simulink model "bf16_mac_new"  (R2022b)
settings: Solver=VariableStepAuto  StartTime=0.0  StopTime=10.0  RelTol=1e-3
libraries: hdlsllib x116, simulink x24
(part 1 of 2)
settings Model: Creator=zishu wu  LastModifiedBy=zishu wu

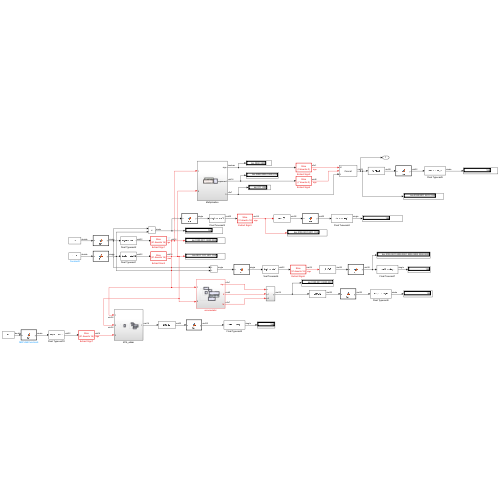
[thumbnail: Simulink's stored preview of the top-level diagram]
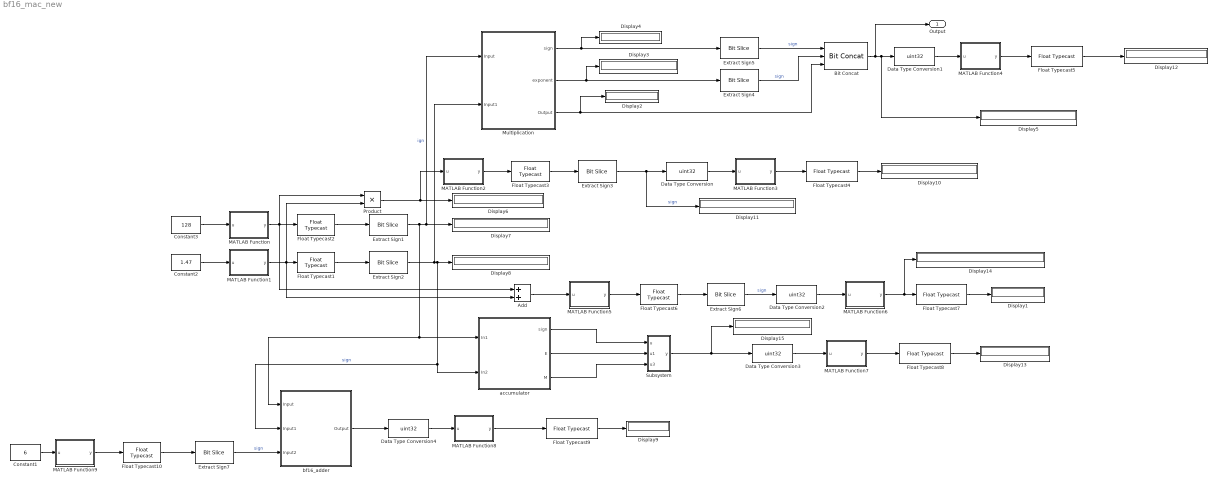
== system bf16_mac_new ==
  Add : Sum
  Bit Concat : hdlsllib/Logic and Bit Operations/Bit Concat  numInputs=3
  Constant1 : Constant  Value=6  OutDataTypeStr=double
  Constant2 : Constant  Value=1.47  OutDataTypeStr=double
  Constant3 : Constant  Value=128  OutDataTypeStr=double  SampleTime=1.5625
  Data Type Conversion{,1..4} (5 alike) : DataTypeConversion  OutDataTypeStr=uint32  SaturateOnIntegerOverflow=off  RndMeth=Floor
  Display{1..15} (15 alike) : Display
      settings: Format=binary (Stored Integer)
  Extract Sign{1..3,6..7} (5 alike) : hdlsllib/Logic and Bit Operations/Bit Slice  lidx=31  ridx=16
  Extract Sign4 : hdlsllib/Logic and Bit Operations/Bit Slice  lidx=7  ridx=0
  Extract Sign5 : hdlsllib/Logic and Bit Operations/Bit Slice  lidx=0  ridx=0
  Float Typecast{1..10} (10 alike) : FloatTypecast
  MATLAB Function : MATLAB Function  TreatAsAtomicUnit=on
  MATLAB Function1 : MATLAB Function  TreatAsAtomicUnit=on
  MATLAB Function2 : MATLAB Function  TreatAsAtomicUnit=on
  MATLAB Function3 : MATLAB Function  TreatAsAtomicUnit=on
  MATLAB Function4 : MATLAB Function  TreatAsAtomicUnit=on
  MATLAB Function5 : MATLAB Function  TreatAsAtomicUnit=on
  MATLAB Function6 : MATLAB Function  TreatAsAtomicUnit=on
  MATLAB Function7 : MATLAB Function  TreatAsAtomicUnit=on
  MATLAB Function8 : MATLAB Function  TreatAsAtomicUnit=on
  MATLAB Function9 : MATLAB Function  TreatAsAtomicUnit=on
  Multiplication : Subsystem
  Product : Product
  Subsystem : Subsystem
  accumulator : Subsystem
  bf16_adder : Subsystem
  Output : Outport
  wires:
  Bit Concat/1 -> Output/1, Display5/1, Data Type Conversion1/1
  Multiplication/2(exponent) -> Extract Sign4/1, Display3/1
  Multiplication/1(sign) -> Display4/1, Extract Sign5/1
  Float Typecast2/1 -> Extract Sign1/1
  MATLAB Function/1(y) -> Add/1, Product/1, Float Typecast2/1
  MATLAB Function1/1(y) -> Add/2, Product/2, Float Typecast1/1
  Float Typecast1/1 -> Extract Sign2/1
  Extract Sign2/1 -> Multiplication/2(Input1), bf16_adder/2(Input1), accumulator/2(In2), Display8/1  "sign"
  Extract Sign1/1 -> Multiplication/1(Input), Display7/1, accumulator/1(In1), bf16_adder/1(Input)  "ign"
  Product/1 -> MATLAB Function2/1(u), Display6/1
  MATLAB Function2/1(y) -> Float Typecast3/1
  Float Typecast3/1 -> Extract Sign3/1
  Extract Sign3/1 -> Display11/1, Data Type Conversion/1  "sign"
  Extract Sign4/1 -> Bit Concat/2  "sign"
  Extract Sign5/1 -> Bit Concat/1  "sign"
  Data Type Conversion/1 -> MATLAB Function3/1(u)
  Float Typecast4/1 -> Display10/1
  Data Type Conversion1/1 -> MATLAB Function4/1(u)
  MATLAB Function3/1(y) -> Float Typecast4/1
  MATLAB Function4/1(y) -> Float Typecast5/1
  Float Typecast6/1 -> Extract Sign6/1
  MATLAB Function5/1(y) -> Float Typecast6/1
  Add/1 -> MATLAB Function5/1(u)
  MATLAB Function6/1(y) -> Display14/1, Float Typecast7/1
  Data Type Conversion2/1 -> MATLAB Function6/1(u)
  Float Typecast7/1 -> Display1/1
  Extract Sign6/1 -> Data Type Conversion2/1  "sign"
  Float Typecast8/1 -> Display13/1
  Data Type Conversion3/1 -> MATLAB Function7/1(u)
  MATLAB Function7/1(y) -> Float Typecast8/1
  Subsystem/1(y) -> Data Type Conversion3/1, Display15/1
  Constant3/1 -> MATLAB Function/1(u)
  Constant2/1 -> MATLAB Function1/1(u)
  Float Typecast5/1 -> Display12/1
  MATLAB Function8/1(y) -> Float Typecast9/1
  Data Type Conversion4/1 -> MATLAB Function8/1(u)
  Float Typecast9/1 -> Display9/1
  bf16_adder/1(Output) -> Data Type Conversion4/1
  accumulator/1(sign) -> Subsystem/1(u)
  accumulator/2(E) -> Subsystem/2(u1)
  accumulator/3(M) -> Subsystem/3(u3)
  Multiplication/3(Output) -> Display2/1, Bit Concat/3
  Float Typecast10/1 -> Extract Sign7/1
  MATLAB Function9/1(y) -> Float Typecast10/1
  Extract Sign7/1 -> bf16_adder/3(Input2)  "sign"
  Constant1/1 -> MATLAB Function9/1(u)

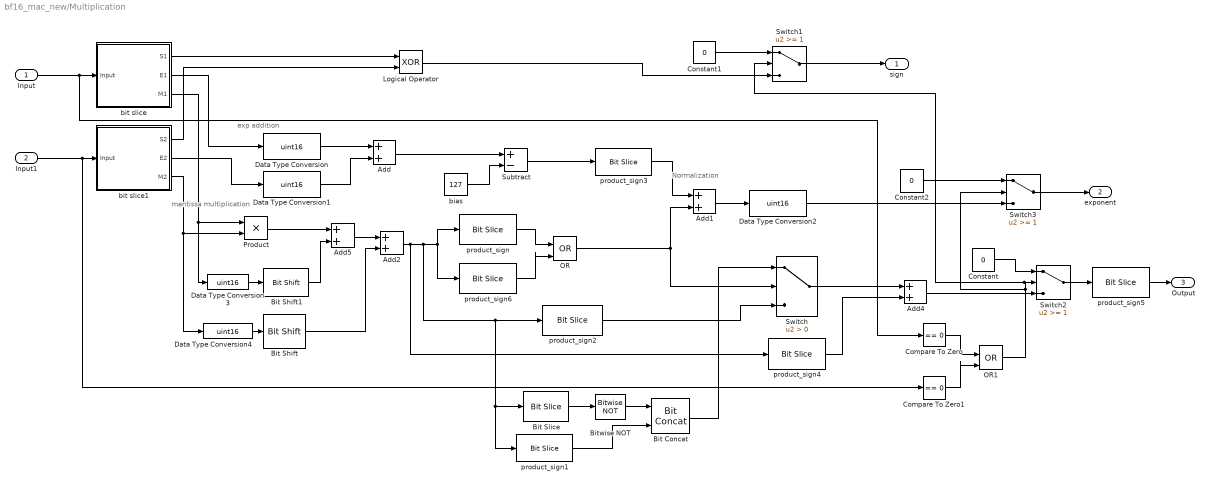
== system bf16_mac_new/Multiplication ==
  note: mantissa multiplication
  note: Normalization
  note: exp addition
  Input : Inport
  Input1 : Inport  Port=2
  Add{,2,4..5} (4 alike) : Sum  AccumDataTypeStr=uint16
  Add1 : Sum
  Bit Concat : hdlsllib/Logic and Bit Operations/Bit Concat  numInputs=2
  Bit Shift : hdlsllib/Logic and Bit Operations/Bit Shift  mode=Shift Left Logical  N=7
  Bit Shift1 : hdlsllib/Logic and Bit Operations/Bit Shift  mode=Shift Left Logical  N=7
  Bit Slice : hdlsllib/Logic and Bit Operations/Bit Slice  lidx=14  ridx=14
  Bitwise NOT : simulink/Logic and Bit Operations/Bitwise Operator  logicop=NOT  UseBitMask=off  BitMask=bin2dec('11011001')  BitMaskRealWorld=Stored Integer
      settings: LibrarySourceBlock=|
      | simulink/Quick Insert/Logic and Bit
      | Operations/Bitwise NOT
  Compare To Zero : simulink/Logic and Bit Operations/Compare To Zero  relop===  OutDataTypeStr=boolean
  Compare To Zero1 : simulink/Logic and Bit Operations/Compare To Zero  relop===  OutDataTypeStr=boolean
  Constant : Constant  Value=0  OutDataTypeStr=uint8
  Constant1 : Constant  Value=0  OutDataTypeStr=boolean
  Constant2 : Constant  Value=0  OutDataTypeStr=uint16
  Data Type Conversion{,1..4} (5 alike) : DataTypeConversion  OutDataTypeStr=uint16  SaturateOnIntegerOverflow=off  RndMeth=Floor
  Logical Operator : Logic  Operator=XOR  AllPortsSameDT=off  OutDataTypeStr=boolean
  OR : Logic  Operator=OR  IconShape=distinctive  AllPortsSameDT=off  OutDataTypeStr=boolean
  OR1 : Logic  Operator=OR  IconShape=distinctive  AllPortsSameDT=off  OutDataTypeStr=boolean
  Product : Product  OutDataTypeStr=uint16
  Subtract : Sum  Inputs=+-
  Switch : Switch  Criteria=u2 > Threshold  SaturateOnIntegerOverflow=off  InputSameDT=off
  Switch1 : Switch  Threshold=1  SaturateOnIntegerOverflow=off  InputSameDT=off
  Switch2 : Switch  Threshold=1  SaturateOnIntegerOverflow=off  InputSameDT=off
  Switch3 : Switch  Threshold=1  SaturateOnIntegerOverflow=off  InputSameDT=off
  bias : Constant  Value=127  OutDataTypeStr=uint16
  bit slice : Subsystem
  bit slice1 : Subsystem
  product_sign : hdlsllib/Logic and Bit Operations/Bit Slice  lidx=15  ridx=15
  product_sign1 : hdlsllib/Logic and Bit Operations/Bit Slice  lidx=13  ridx=7
  product_sign2 : hdlsllib/Logic and Bit Operations/Bit Slice  lidx=13  ridx=6
  product_sign3 : hdlsllib/Logic and Bit Operations/Bit Slice  lidx=7  ridx=0
  product_sign4 : hdlsllib/Logic and Bit Operations/Bit Slice  lidx=0  ridx=0
  product_sign5 : hdlsllib/Logic and Bit Operations/Bit Slice  lidx=7  ridx=1
  product_sign6 : hdlsllib/Logic and Bit Operations/Bit Slice  lidx=14  ridx=14
  sign : Outport
  exponent : Outport  Port=2
  Output : Outport  Port=3
  wires:
  product_sign/1 -> OR/1
  Compare To Zero1/1 -> OR1/2
  Bitwise NOT/1 -> Bit Concat/1
  Add5/1 -> Add2/1
  Input/1 -> Compare To Zero/1, bit slice/1(Input)
  Product/1 -> Add5/1
  product_sign6/1 -> OR/2
  Switch/1 -> Add4/1
  Subtract/1 -> product_sign3/1
  Data Type Conversion4/1 -> Bit Shift/1
  bit slice1/1(S2) -> Logical Operator/2
  Input1/1 -> Compare To Zero1/1, bit slice1/1(Input)
  Add1/1 -> Data Type Conversion2/1
  Constant2/1 -> Switch3/1
  Switch1/1 -> sign/1
  Data Type Conversion/1 -> Add/1
  Bit Slice/1 -> Bitwise NOT/1
  Switch3/1 -> exponent/1
  product_sign3/1 -> Add1/1
  OR1/1 -> Switch1/2, Switch2/2, Switch3/2
  Constant1/1 -> Switch1/1
  Data Type Conversion1/1 -> Add/2
  Constant/1 -> Switch2/1
  Add2/1 -> product_sign4/1, product_sign1/1, Bit Slice/1, product_sign2/1, product_sign6/1, product_sign/1
  product_sign5/1 -> Output/1
  product_sign4/1 -> Add4/2
  Logical Operator/1 -> Switch1/3
  Bit Concat/1 -> Switch/1
  bias/1 -> Subtract/2
  Data Type Conversion2/1 -> Switch3/3
  OR/1 -> Add1/2, Switch/2
  Switch2/1 -> product_sign5/1
  bit slice/2(E1) -> Data Type Conversion/1
  Add4/1 -> Switch2/3
  Compare To Zero/1 -> OR1/1
  product_sign2/1 -> Switch/3
  product_sign1/1 -> Bit Concat/2
  bit slice/3(M1) -> Data Type Conversion3/1, Product/1
  Bit Shift/1 -> Add2/2
  bit slice1/2(E2) -> Data Type Conversion1/1
  Bit Shift1/1 -> Add5/2
  bit slice1/3(M2) -> Data Type Conversion4/1, Product/2
  bit slice/1(S1) -> Logical Operator/1
  Data Type Conversion3/1 -> Bit Shift1/1
  Add/1 -> Subtract/1

== system bf16_mac_new/Subsystem ==
  u : Inport
  u1 : Inport  Port=2
  u3 : Inport  Port=3
  Bit Concat1 : hdlsllib/Logic and Bit Operations/Bit Concat  numInputs=3
  Extract Sign6 : hdlsllib/Logic and Bit Operations/Bit Slice  lidx=7  ridx=0
  Extract Sign7 : hdlsllib/Logic and Bit Operations/Bit Slice  lidx=0  ridx=0
  y : Outport
  wires:
  u/1 -> Extract Sign7/1
  u3/1 -> Bit Concat1/3
  Extract Sign7/1 -> Bit Concat1/1  "sign"
  Extract Sign6/1 -> Bit Concat1/2  "sign"
  u1/1 -> Extract Sign6/1
  Bit Concat1/1 -> y/1

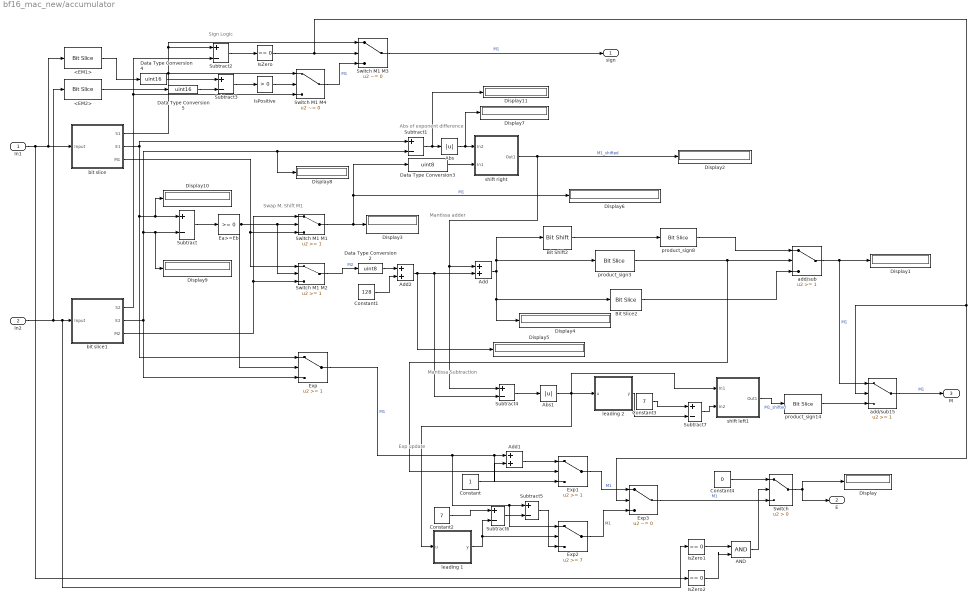
== system bf16_mac_new/accumulator ==
  note: Mantissa Subtraction
  note: Exp update
  note: Mantissa adder
  note: Sign Logic
  note: Abs of exponent difference
  note: Swap M, Shift M1
  In1 : Inport
  In2 : Inport  Port=2
  <EM1> : hdlsllib/Logic and Bit Operations/Bit Slice  lidx=14  ridx=0
  <EM2> : hdlsllib/Logic and Bit Operations/Bit Slice  lidx=14  ridx=0
  AND : Logic  IconShape=distinctive  AllPortsSameDT=off  OutDataTypeStr=boolean
  Abs : Abs  SaturateOnIntegerOverflow=off
  Abs1 : Abs  SaturateOnIntegerOverflow=off
  Add : Sum  OutDataTypeStr=uint16
  Add1 : Sum
  Add2 : Sum
  Bit Shift2 : hdlsllib/Logic and Bit Operations/Bit Shift  mode=Shift Right Logical  N=1
  Bit Slice2 : hdlsllib/Logic and Bit Operations/Bit Slice  lidx=6  ridx=0
  Constant : Constant  OutDataTypeStr=uint8
  Constant1 : Constant  Value=128  OutDataTypeStr=uint8
  Constant2 : Constant  Value=7
  Constant3 : Constant  Value=7
  Constant4 : Constant  Value=0  OutDataTypeStr=uint8
  Data Type Conversion2 : DataTypeConversion  OutDataTypeStr=uint8  SaturateOnIntegerOverflow=off  RndMeth=Floor
  Data Type Conversion3 : DataTypeConversion  OutDataTypeStr=uint8  SaturateOnIntegerOverflow=off  RndMeth=Floor
  Data Type Conversion4 : DataTypeConversion  OutDataTypeStr=uint16  SaturateOnIntegerOverflow=off  RndMeth=Floor
  Data Type Conversion5 : DataTypeConversion  OutDataTypeStr=uint16  SaturateOnIntegerOverflow=off  RndMeth=Floor
  Display{,1..11} (12 alike) : Display
      Display settings: Format=binary (Stored Integer)
      Display1 settings: Format=binary (Stored Integer)
      Display10 settings: Format=binary (Stored Integer)
      Display11 settings: Format=decimal (Stored Integer)
      Display2 settings: Format=binary (Stored Integer)
      Display3 settings: Format=binary (Stored Integer)
      Display4 settings: Format=binary (Stored Integer)
      Display5 settings: Format=binary (Stored Integer)
      Display6 settings: Format=binary (Stored Integer)
      Display7 settings: Format=decimal (Stored Integer)
      Display8 settings: Format=binary (Stored Integer)
      Display9 settings: Format=binary (Stored Integer)
  Ea>=Eb : hdlsllib/Logic and Bit Operations/Compare To Zero  relop=>=  OutDataTypeStr=boolean
  Exp : Switch  Threshold=1  SaturateOnIntegerOverflow=off  InputSameDT=off
  Exp1 : Switch  Threshold=1  SaturateOnIntegerOverflow=off  InputSameDT=off
  Exp2 : Switch  Threshold=7  SaturateOnIntegerOverflow=off  InputSameDT=off
  Exp3 : Switch  Criteria=u2 ~= 0  Threshold=1  SaturateOnIntegerOverflow=off  InputSameDT=off
  IsPositive : simulink/Logic and Bit Operations/Compare To Zero  relop=>  OutDataTypeStr=boolean
      settings: LibrarySourceBlock=|
      | simulink/Quick Insert/Logic and Bit
      | Operations/IsPositive
  IsZero : simulink/Logic and Bit Operations/Compare To Zero  relop===  OutDataTypeStr=boolean
      settings: LibrarySourceBlock=|
      | simulink/Quick Insert/Logic and Bit
      | Operations/IsZero
  IsZero1 : simulink/Logic and Bit Operations/Compare To Zero  relop===  OutDataTypeStr=boolean
      settings: LibrarySourceBlock=|
      | simulink/Quick Insert/Logic and Bit
      | Operations/IsZero
  IsZero2 : simulink/Logic and Bit Operations/Compare To Zero  relop===  OutDataTypeStr=boolean
      settings: LibrarySourceBlock=|
      | simulink/Quick Insert/Logic and Bit
      | Operations/IsZero
  Subtract{,1,3..4} (4 alike) : Sum  Inputs=+-  OutDataTypeStr=int16
  Subtract2 : Sum  Inputs=+-  OutDataTypeStr=int8
  Subtract5 : Sum  Inputs=+-  OutDataTypeStr=uint8
  Subtract6 : Sum  Inputs=+-  OutDataTypeStr=uint8
  Subtract7 : Sum  Inputs=+-  OutDataTypeStr=uint8
  Switch : Switch  Criteria=u2 > Threshold  SaturateOnIntegerOverflow=off  InputSameDT=off
  Switch M1 M1 : Switch  Threshold=1  SaturateOnIntegerOverflow=off  InputSameDT=off
  Switch M1 M2 : Switch  Threshold=1  SaturateOnIntegerOverflow=off  InputSameDT=off
  Switch M1 M3 : Switch  Criteria=u2 ~= 0  Threshold=1  SaturateOnIntegerOverflow=off  InputSameDT=off
  Switch M1 M4 : Switch  Criteria=u2 ~= 0  Threshold=1  SaturateOnIntegerOverflow=off  InputSameDT=off
  add/sub : Switch  Threshold=1  SaturateOnIntegerOverflow=off  InputSameDT=off
  add/sub15 : Switch  Threshold=1  SaturateOnIntegerOverflow=off  InputSameDT=off
  bit slice : Subsystem
  bit slice1 : Subsystem
  leading 1 : Subsystem
  leading 2 : Subsystem
  product_sign14 : hdlsllib/Logic and Bit Operations/Bit Slice  lidx=6  ridx=0
  product_sign3 : hdlsllib/Logic and Bit Operations/Bit Slice  lidx=8  ridx=8
  product_sign8 : hdlsllib/Logic and Bit Operations/Bit Slice  lidx=6  ridx=0
  shift left1 : Subsystem
  shift right : Subsystem
  sign : Outport
  E : Outport  Port=2
  M : Outport  Port=3
  wires:
  In1/1 -> bit slice/1(Input), <EM1>/1, IsZero2/1
  Subtract/1 -> Ea>=Eb/1
  Ea>=Eb/1 -> Exp/2, Switch M1 M2/2, Switch M1 M1/2
  bit slice/3(M1) -> Switch M1 M1/3, Switch M1 M2/1
  bit slice1/3(M2) -> Switch M1 M2/3, Switch M1 M1/1
  Switch M1 M1/1 -> Display6/1, Data Type Conversion3/1, Display3/1  "M1"
  Subtract1/1 -> Display11/1, Abs/1
  bit slice1/1(S2) -> Switch M1 M4/3, Subtract2/2
  bit slice/1(S1) -> Switch M1 M4/1, Subtract2/1, Switch M1 M3/1
  Subtract2/1 -> IsZero/1
  IsZero/1 -> add/sub15/2, Exp3/2, Switch M1 M3/2
  Abs/1 -> Display7/1, shift right/1(In2)
  shift right/1(Out1) -> Subtract4/1, Add/1, Display2/1  "M1_shifted"
  IsPositive/1 -> Switch M1 M4/2
  Switch M1 M4/1 -> Switch M1 M3/3  "M1"
  Switch M1 M3/1 -> sign/1  "M1"
  Switch M1 M2/1 -> Data Type Conversion2/1  "M2"
  Subtract3/1 -> IsPositive/1
  <EM1>/1 -> Data Type Conversion4/1
  <EM2>/1 -> Data Type Conversion5/1
  Subtract4/1 -> Abs1/1
  Data Type Conversion3/1 -> shift right/2(In1)
  Data Type Conversion2/1 -> Add2/1
  add/sub/1 -> add/sub15/1, Display1/1  "M1"
  Exp/1 -> Exp2/1, Subtract5/1, Add1/1, Exp1/3  "M1"
  product_sign3/1 -> add/sub/2, Exp1/2
  Constant/1 -> Add1/2
  Add1/1 -> Exp1/1
  Subtract5/1 -> Exp2/3
  Add/1 -> Bit Slice2/1, Display4/1, product_sign3/1, Bit Shift2/1
  Bit Shift2/1 -> product_sign8/1
  Bit Slice2/1 -> add/sub/3
  Add2/1 -> Subtract4/2, Add/2, Display5/1
  Constant1/1 -> Add2/2
  product_sign8/1 -> add/sub/1
  product_sign14/1 -> add/sub15/3
  Exp1/1 -> Exp3/1  "M1"
  Exp2/1 -> Exp3/3  "M1"
  Data Type Conversion4/1 -> Subtract3/1
  Data Type Conversion5/1 -> Subtract3/2
  add/sub15/1 -> M/1  "M1"
  leading 1/1(y) -> Subtract6/2, Exp2/2
  Constant2/1 -> Subtract6/1
  Subtract6/1 -> Subtract5/2
  leading 2/1(y) -> Subtract7/2
  Constant3/1 -> Subtract7/1
  Abs1/1 -> leading 1/1(u), shift left1/1(In1), leading 2/1(u)
  Subtract7/1 -> shift left1/2(In2)
  shift left1/1(Out1) -> product_sign14/1  "M1_shifted"
  bit slice/2(E1) -> Subtract1/1, Display10/1, Subtract/1, Exp/1
  bit slice1/2(E2) -> Exp/3, Display9/1, Subtract/2, Display8/1, Subtract1/2
  Switch/1 -> E/1, Display/1
  IsZero1/1 -> AND/1
  IsZero2/1 -> AND/2
  AND/1 -> Switch/2
  In2/1 -> bit slice1/1(Input), IsZero1/1, <EM2>/1
  Exp3/1 -> Switch/3  "M1"
  Constant4/1 -> Switch/1

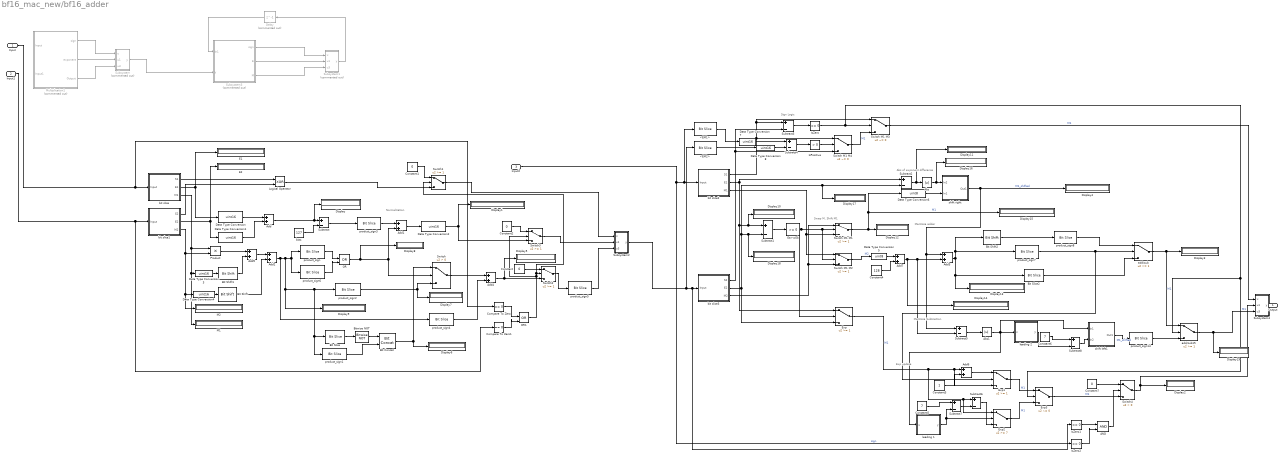
== system bf16_mac_new/bf16_adder ==
  note: Normalization
  note: Exp update
  note: Mantissa adder
  note: Swap M, Shift M1
  note: Abs of exponent difference
  note: Mantissa Subtraction
  note: Sign Logic
  Input : Inport  OutDataTypeStr=uint16
  Input1 : Inport  Port=2  OutDataTypeStr=uint16
  Input2 : Inport  Port=3
  <EM1> : hdlsllib/Logic and Bit Operations/Bit Slice  lidx=14  ridx=0
  <EM2> : hdlsllib/Logic and Bit Operations/Bit Slice  lidx=14  ridx=0
  AND : Logic  IconShape=distinctive  AllPortsSameDT=off  OutDataTypeStr=boolean
  Abs : Abs  SaturateOnIntegerOverflow=off
  Abs1 : Abs  SaturateOnIntegerOverflow=off
  Add{,2,4..5} (4 alike) : Sum  AccumDataTypeStr=uint16
  Add1 : Sum
  Add3 : Sum  OutDataTypeStr=uint16
  Add6 : Sum
  Add7 : Sum
  Bit Concat : hdlsllib/Logic and Bit Operations/Bit Concat  numInputs=2
  Bit Shift : hdlsllib/Logic and Bit Operations/Bit Shift  mode=Shift Left Logical  N=7
  Bit Shift1 : hdlsllib/Logic and Bit Operations/Bit Shift  mode=Shift Left Logical  N=7
  Bit Shift2 : hdlsllib/Logic and Bit Operations/Bit Shift  mode=Shift Right Logical  N=1
  Bit Slice : hdlsllib/Logic and Bit Operations/Bit Slice  lidx=14  ridx=14
  Bit Slice2 : hdlsllib/Logic and Bit Operations/Bit Slice  lidx=6  ridx=0
  Bitwise NOT : simulink/Logic and Bit Operations/Bitwise Operator  logicop=NOT  UseBitMask=off  BitMask=bin2dec('11011001')  BitMaskRealWorld=Stored Integer
      settings: LibrarySourceBlock=|
      | simulink/Quick Insert/Logic and Bit
      | Operations/Bitwise NOT
  Compare To Zero : simulink/Logic and Bit Operations/Compare To Zero  relop===  OutDataTypeStr=boolean
  Compare To Zero1 : simulink/Logic and Bit Operations/Compare To Zero  relop===  OutDataTypeStr=boolean
  Constant : Constant  Value=0  OutDataTypeStr=uint8
  Constant1 : Constant  Value=0  OutDataTypeStr=boolean
  Constant2 : Constant  Value=0  OutDataTypeStr=uint16
  Constant3 : Constant  OutDataTypeStr=uint8
  Constant4 : Constant  Value=128  OutDataTypeStr=uint8
  Constant5 : Constant  Value=7
  Constant6 : Constant  Value=7
  Constant7 : Constant  Value=0  OutDataTypeStr=uint8
  Data Type Conversion{,1..4,7..8} (7 alike) : DataTypeConversion  OutDataTypeStr=uint16  SaturateOnIntegerOverflow=off  RndMeth=Floor
  Data Type Conversion5 : DataTypeConversion  OutDataTypeStr=uint8  SaturateOnIntegerOverflow=off  RndMeth=Floor
  Data Type Conversion6 : DataTypeConversion  OutDataTypeStr=uint8  SaturateOnIntegerOverflow=off  RndMeth=Floor
  Delay : Delay  Commented=on  DelayLength=1
  Display{,1..19} (20 alike) : Display
      Display settings: Format=binary (Stored Integer)
      Display1 settings: Format=binary (Stored Integer)
      Display10 settings: Format=binary (Stored Integer)
      Display11 settings: Format=decimal (Stored Integer)
      Display12 settings: Format=binary (Stored Integer)
      Display13 settings: Format=binary (Stored Integer)
      Display14 settings: Format=binary (Stored Integer)
      Display15 settings: Format=binary (Stored Integer)
      Display16 settings: Format=decimal (Stored Integer)
      Display17 settings: Format=binary (Stored Integer)
      Display18 settings: Format=binary (Stored Integer)
      Display19 settings: Format=binary (Stored Integer)
      Display2 settings: Format=binary (Stored Integer)
      Display3 settings: Format=binary (Stored Integer)
      Display4 settings: Format=binary (Stored Integer)
      Display5 settings: Format=binary (Stored Integer)
      Display6 settings: Format=binary (Stored Integer)
      Display7 settings: Format=binary (Stored Integer)
      Display8 settings: Format=binary (Stored Integer)
      Display9 settings: Format=binary (Stored Integer)
  E1 : Display
      settings: Format=binary (Stored Integer)
  E2 : Display
      settings: Format=binary (Stored Integer)
  Ea>=Eb : hdlsllib/Logic and Bit Operations/Compare To Zero  relop=>=  OutDataTypeStr=boolean
  Exp : Switch  Threshold=1  SaturateOnIntegerOverflow=off  InputSameDT=off
  Exp1 : Switch  Threshold=1  SaturateOnIntegerOverflow=off  InputSameDT=off
  Exp2 : Switch  Threshold=7  SaturateOnIntegerOverflow=off  InputSameDT=off
  Exp3 : Switch  Criteria=u2 ~= 0  Threshold=1  SaturateOnIntegerOverflow=off  InputSameDT=off
  IsPositive : simulink/Logic and Bit Operations/Compare To Zero  relop=>  OutDataTypeStr=boolean
      settings: LibrarySourceBlock=|
      | simulink/Quick Insert/Logic and Bit
      | Operations/IsPositive
  IsZero : simulink/Logic and Bit Operations/Compare To Zero  relop===  OutDataTypeStr=boolean
      settings: LibrarySourceBlock=|
      | simulink/Quick Insert/Logic and Bit
      | Operations/IsZero
  IsZero1 : simulink/Logic and Bit Operations/Compare To Zero  relop===  OutDataTypeStr=boolean
      settings: LibrarySourceBlock=|
      | simulink/Quick Insert/Logic and Bit
      | Operations/IsZero
  IsZero2 : simulink/Logic and Bit Operations/Compare To Zero  relop===  OutDataTypeStr=boolean
      settings: LibrarySourceBlock=|
      | simulink/Quick Insert/Logic and Bit
      | Operations/IsZero
  Logical Operator : Logic  Operator=XOR  AllPortsSameDT=off  OutDataTypeStr=boolean
  M1 : Display
      settings: Format=binary (Stored Integer)
  M2 : Display
      settings: Format=binary (Stored Integer)
  Multiplication1 : Subsystem  Commented=on
  OR : Logic  Operator=OR  IconShape=distinctive  AllPortsSameDT=off  OutDataTypeStr=boolean
  OR1 : Logic  Operator=OR  IconShape=distinctive  AllPortsSameDT=off  OutDataTypeStr=boolean
  Product : Product  OutDataTypeStr=uint16
  Subsystem : Subsystem  Commented=on
  Subsystem1 : Subsystem  Commented=on
  Subsystem2 : Subsystem
  Subsystem3 : Subsystem  Commented=on
  Subsystem4 : Subsystem
  Subtract : Sum  Inputs=+-
  Subtract{1..2,4..5} (4 alike) : Sum  Inputs=+-  OutDataTypeStr=int16
  Subtract3 : Sum  Inputs=+-  OutDataTypeStr=int8
  Subtract6 : Sum  Inputs=+-  OutDataTypeStr=uint8
  Subtract7 : Sum  Inputs=+-  OutDataTypeStr=uint8
  Subtract8 : Sum  Inputs=+-  OutDataTypeStr=uint8
  Switch : Switch  Criteria=u2 > Threshold  SaturateOnIntegerOverflow=off  InputSameDT=off
  Switch M1 M1 : Switch  Threshold=1  SaturateOnIntegerOverflow=off  InputSameDT=off
  Switch M1 M2 : Switch  Threshold=1  SaturateOnIntegerOverflow=off  InputSameDT=off
  Switch M1 M3 : Switch  Criteria=u2 ~= 0  Threshold=1  SaturateOnIntegerOverflow=off  InputSameDT=off
  Switch M1 M4 : Switch  Criteria=u2 ~= 0  Threshold=1  SaturateOnIntegerOverflow=off  InputSameDT=off
  Switch1 : Switch  Threshold=1  SaturateOnIntegerOverflow=off  InputSameDT=off
  Switch2 : Switch  Threshold=1  SaturateOnIntegerOverflow=off  InputSameDT=off
  Switch3 : Switch  Threshold=1  SaturateOnIntegerOverflow=off  InputSameDT=off
  Switch4 : Switch  Criteria=u2 > Threshold  SaturateOnIntegerOverflow=off  InputSameDT=off
  add/sub : Switch  Threshold=1  SaturateOnIntegerOverflow=off  InputSameDT=off
  add/sub15 : Switch  Threshold=1  SaturateOnIntegerOverflow=off  InputSameDT=off
  bias : Constant  Value=127  OutDataTypeStr=uint16
  bit slice : Subsystem
  bit slice1 : Subsystem
  bit slice2 : Subsystem
  bit slice3 : Subsystem
  leading 1 : Subsystem
  leading 2 : Subsystem
  product_sign : hdlsllib/Logic and Bit Operations/Bit Slice  lidx=15  ridx=15
  product_sign1 : hdlsllib/Logic and Bit Operations/Bit Slice  lidx=13  ridx=7
  product_sign14 : hdlsllib/Logic and Bit Operations/Bit Slice  lidx=6  ridx=0
  product_sign2 : hdlsllib/Logic and Bit Operations/Bit Slice  lidx=13  ridx=6
  product_sign3 : hdlsllib/Logic and Bit Operations/Bit Slice  lidx=7  ridx=0
  product_sign4 : hdlsllib/Logic and Bit Operations/Bit Slice  lidx=0  ridx=0
  product_sign5 : hdlsllib/Logic and Bit Operations/Bit Slice  lidx=7  ridx=1
  product_sign6 : hdlsllib/Logic and Bit Operations/Bit Slice  lidx=14  ridx=14
  product_sign7 : hdlsllib/Logic and Bit Operations/Bit Slice  lidx=8  ridx=8
  product_sign8 : hdlsllib/Logic and Bit Operations/Bit Slice  lidx=6  ridx=0
  shift left1 : Subsystem
  shift right : Subsystem
  Output : Outport
  wires:
  Subsystem1/1(y) -> Delay/1
  Subsystem/1(y) -> Subsystem3/2(y)
  Multiplication1/3(Output) -> Subsystem/3(u3)
  Multiplication1/2(exponent) -> Subsystem/2(u1)
  Multiplication1/1(sign) -> Subsystem/1(u)
  Subsystem3/3(M) -> Subsystem1/3(u3)
  Subsystem3/2(E) -> Subsystem1/2(u1)
  Subsystem3/1(sign) -> Subsystem1/1(u)
  Delay/1 -> Subsystem3/1(In1)
  Switch1/1 -> Subsystem2/1(u)
  bit slice/1(S1) -> Logical Operator/1
  Switch2/1 -> product_sign5/1
  Subtract/1 -> product_sign3/1
  product_sign1/1 -> Bit Concat/2
  Data Type Conversion2/1 -> Display1/1, Switch3/3
  bias/1 -> Subtract/2
  product_sign2/1 -> Switch/3, Display7/1
  Data Type Conversion1/1 -> Add/2
  Data Type Conversion/1 -> Add/1
  Add2/1 -> product_sign4/1, product_sign1/1, Bit Slice/1, product_sign2/1, Display9/1, product_sign6/1, product_sign/1
  Bit Shift/1 -> Add2/2
  Input1/1 -> Compare To Zero1/1, bit slice1/1(Input)
  product_sign4/1 -> Add4/2
  Bitwise NOT/1 -> Bit Concat/1
  Logical Operator/1 -> Switch1/3
  Add1/1 -> Data Type Conversion2/1
  Add/1 -> Display/1, Subtract/1
  Input/1 -> Compare To Zero/1, bit slice/1(Input)
  Constant1/1 -> Switch1/1
  Constant2/1 -> Switch3/1
  bit slice/3(M1) -> Data Type Conversion3/1, M1/1, Product/1
  Bit Slice/1 -> Bitwise NOT/1
  Switch3/1 -> Subsystem2/2(u1)
  bit slice/2(E1) -> Data Type Conversion/1, E1/1
  Add5/1 -> Add2/1
  OR1/1 -> Switch1/2, Switch2/2, Switch3/2
  product_sign/1 -> OR/1
  Switch/1 -> Add4/1
  bit slice1/3(M2) -> Data Type Conversion4/1, M2/1, Product/2
  Compare To Zero/1 -> OR1/1
  Add4/1 -> Display5/1, Switch2/3
  bit slice1/1(S2) -> Logical Operator/2
  Data Type Conversion4/1 -> Bit Shift/1
  product_sign3/1 -> Add1/1
  Bit Shift1/1 -> Add5/2
  Data Type Conversion3/1 -> Bit Shift1/1
  Compare To Zero1/1 -> OR1/2
  product_sign5/1 -> Subsystem2/3(u3)
  Bit Concat/1 -> Switch/1, Display6/1
  OR/1 -> Add1/2, Switch/2, Display8/1
  product_sign6/1 -> OR/2
  Product/1 -> Add5/1
  bit slice1/2(E2) -> Data Type Conversion1/1, E2/1
  Constant/1 -> Switch2/1
  Switch M1 M2/1 -> Data Type Conversion5/1  "M2"
  leading 1/1(y) -> Subtract7/2, Exp2/2
  Add3/1 -> Bit Slice2/1, Display13/1, product_sign7/1, Bit Shift2/1
  Constant7/1 -> Switch4/1
  bit slice3/2(E2) -> Exp/3, Display18/1, Subtract1/2, Display17/1, Subtract2/2
  bit slice3/1(S2) -> Switch M1 M4/3, Subtract3/2
  Data Type Conversion7/1 -> Subtract4/1
  IsZero2/1 -> AND/2
  bit slice2/2(E1) -> Subtract2/1, Display10/1, Subtract1/1, Exp/1
  IsZero1/1 -> AND/1
  Data Type Conversion8/1 -> Subtract4/2
  <EM1>/1 -> Data Type Conversion7/1
  product_sign14/1 -> add/sub15/3
  Switch4/1 -> Subsystem4/2(u1), Display2/1
  AND/1 -> Switch4/2
  add/sub15/1 -> Display19/1, Subsystem4/3(u3)  "M1"
  shift left1/1(Out1) -> product_sign14/1  "M1_shifted"
  Subtract7/1 -> Subtract6/2
  Subtract8/1 -> shift left1/2(In2)
  Constant5/1 -> Subtract7/1
  Ea>=Eb/1 -> Exp/2, Switch M1 M2/2, Switch M1 M1/2
  Constant6/1 -> Subtract8/1
  Switch M1 M4/1 -> Switch M1 M3/3  "M1"
  Subtract6/1 -> Exp2/3
  bit slice3/3(M2) -> Switch M1 M2/3, Switch M1 M1/1
  Add6/1 -> Exp1/1
  Subtract4/1 -> IsPositive/1
  product_sign8/1 -> add/sub/1
  Constant3/1 -> Add6/2
  Exp/1 -> Exp2/1, Subtract6/1, Add6/1, Exp1/3  "M1"
  Bit Shift2/1 -> product_sign8/1
  bit slice2/3(M1) -> Switch M1 M1/3, Switch M1 M2/1
  Data Type Conversion6/1 -> shift right/2(In1)
  <EM2>/1 -> Data Type Conversion8/1
  product_sign7/1 -> add/sub/2, Exp1/2
  IsPositive/1 -> Switch M1 M4/2
  shift right/1(Out1) -> Subtract5/1, Add3/1, Display4/1  "M1_shifted"
  Subtract3/1 -> IsZero/1
  IsZero/1 -> add/sub15/2, Exp3/2, Switch M1 M3/2
  bit slice2/1(S1) -> Switch M1 M4/1, Subtract3/1, Switch M1 M3/1
  Subtract1/1 -> Ea>=Eb/1
  Exp1/1 -> Exp3/1  "M1"
  Exp2/1 -> Exp3/3  "M1"
  Abs1/1 -> leading 1/1(u), shift left1/1(In1), leading 2/1(u)
  Subsystem2/1(y) -> bit slice3/1(Input), IsZero1/1, <EM2>/1
  Data Type Conversion5/1 -> Add7/1
  leading 2/1(y) -> Subtract8/2
  Exp3/1 -> Switch4/3  "M1"
  Abs/1 -> Display16/1, shift right/1(In2)
  Switch M1 M3/1 -> Subsystem4/1(u)  "M1"
  Add7/1 -> Subtract5/2, Add3/2, Display14/1
  Constant4/1 -> Add7/2
  Switch M1 M1/1 -> Display15/1, Data Type Conversion6/1, Display12/1  "M1"
  Subtract2/1 -> Display11/1, Abs/1
  add/sub/1 -> add/sub15/1, Display3/1  "M1"
  Bit Slice2/1 -> add/sub/3
  Subtract5/1 -> Abs1/1
  Subsystem4/1(y) -> Output/1
  Input2/1 -> IsZero2/1, bit slice2/1(Input), <EM1>/1  "sign"

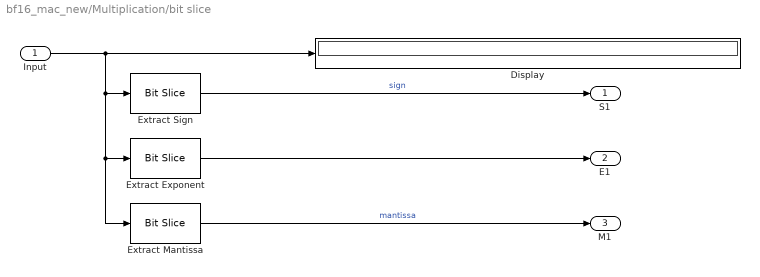
== system bf16_mac_new/Multiplication/bit slice ==
  Input : Inport
  Display : Display
      settings: Format=binary (Stored Integer)
  Extract Exponent : hdlsllib/Logic and Bit Operations/Bit Slice  lidx=14  ridx=7
  Extract Mantissa : hdlsllib/Logic and Bit Operations/Bit Slice  lidx=6  ridx=0
  Extract Sign : hdlsllib/Logic and Bit Operations/Bit Slice  lidx=15  ridx=15
  S1 : Outport
  E1 : Outport  Port=2
  M1 : Outport  Port=3
  wires:
  Input/1 -> Extract Mantissa/1, Extract Exponent/1, Extract Sign/1, Display/1
  Extract Mantissa/1 -> M1/1  "mantissa"
  Extract Sign/1 -> S1/1  "sign"
  Extract Exponent/1 -> E1/1

== system bf16_mac_new/Multiplication/bit slice1 ==
  Input : Inport
  Extract Exponent : hdlsllib/Logic and Bit Operations/Bit Slice  lidx=14  ridx=7
  Extract Mantissa : hdlsllib/Logic and Bit Operations/Bit Slice  lidx=6  ridx=0
  Extract Sign : hdlsllib/Logic and Bit Operations/Bit Slice  lidx=15  ridx=15
  S2 : Outport
  E2 : Outport  Port=2
  M2 : Outport  Port=3
  wires:
  Input/1 -> Extract Mantissa/1, Extract Exponent/1, Extract Sign/1
  Extract Mantissa/1 -> M2/1  "mantissa"
  Extract Sign/1 -> S2/1  "sign"
  Extract Exponent/1 -> E2/1

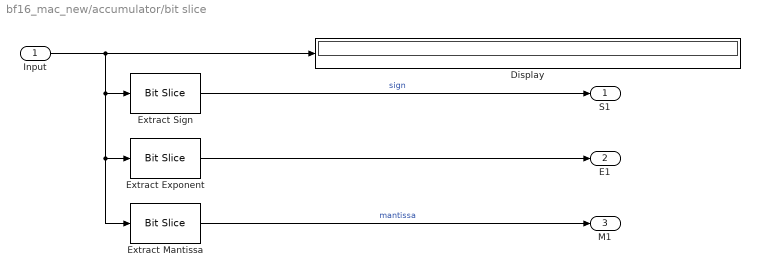
== system bf16_mac_new/accumulator/bit slice ==
  Input : Inport
  Display : Display
      settings: Format=binary (Stored Integer)
  Extract Exponent : hdlsllib/Logic and Bit Operations/Bit Slice  lidx=14  ridx=7
  Extract Mantissa : hdlsllib/Logic and Bit Operations/Bit Slice  lidx=6  ridx=0
  Extract Sign : hdlsllib/Logic and Bit Operations/Bit Slice  lidx=15  ridx=15
  S1 : Outport
  E1 : Outport  Port=2
  M1 : Outport  Port=3
  wires:
  Input/1 -> Extract Mantissa/1, Extract Exponent/1, Extract Sign/1, Display/1
  Extract Mantissa/1 -> M1/1  "mantissa"
  Extract Sign/1 -> S1/1  "sign"
  Extract Exponent/1 -> E1/1

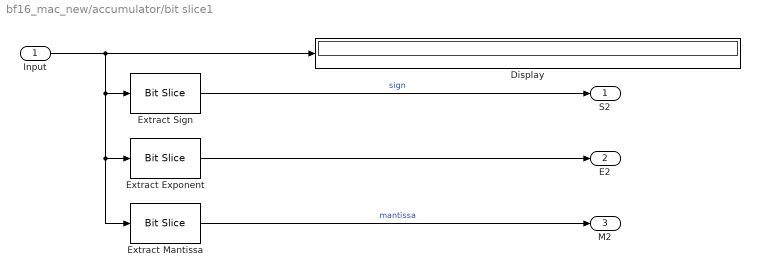
== system bf16_mac_new/accumulator/bit slice1 ==
  Input : Inport
  Display : Display
      settings: Format=binary (Stored Integer)
  Extract Exponent : hdlsllib/Logic and Bit Operations/Bit Slice  lidx=14  ridx=7
  Extract Mantissa : hdlsllib/Logic and Bit Operations/Bit Slice  lidx=6  ridx=0
  Extract Sign : hdlsllib/Logic and Bit Operations/Bit Slice  lidx=15  ridx=15
  S2 : Outport
  E2 : Outport  Port=2
  M2 : Outport  Port=3
  wires:
  Input/1 -> Extract Mantissa/1, Extract Exponent/1, Extract Sign/1, Display/1
  Extract Mantissa/1 -> M2/1  "mantissa"
  Extract Sign/1 -> S2/1  "sign"
  Extract Exponent/1 -> E2/1

== system bf16_mac_new/accumulator/leading 1 ==
  u : Inport
  MATLAB Function : MATLAB Function  TreatAsAtomicUnit=on
  y : Outport
  wires:
  u/1 -> MATLAB Function/1(u)
  MATLAB Function/1(y) -> y/1

== system bf16_mac_new/accumulator/leading 2 ==
  u : Inport
  MATLAB Function : MATLAB Function  TreatAsAtomicUnit=on
  y : Outport
  wires:
  u/1 -> MATLAB Function/1(u)
  MATLAB Function/1(y) -> y/1

== system bf16_mac_new/accumulator/shift left1 ==
  In1 : Inport
  In2 : Inport  Port=2
  Constant : Constant  Value=2  OutDataTypeStr=half
  Data Type Conversion1 : DataTypeConversion  OutDataTypeStr=uint8  SaturateOnIntegerOverflow=off  RndMeth=Floor
  Data Type Conversion2 : DataTypeConversion  OutDataTypeStr=half  SaturateOnIntegerOverflow=off  RndMeth=Floor
  Pow : Math  Operator=pow  SignedPower=on  RndMeth=Zero
  Product : Product
  Out1 : Outport
  wires:
  Pow/1 -> Data Type Conversion1/1
  Constant/1 -> Pow/1
  In2/1 -> Data Type Conversion2/1
  Product/1 -> Out1/1
  Data Type Conversion1/1 -> Product/2
  Data Type Conversion2/1 -> Pow/2
  In1/1 -> Product/1

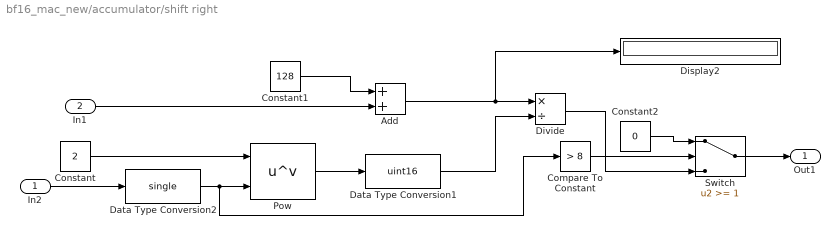
== system bf16_mac_new/accumulator/shift right ==
  In2 : Inport
  In1 : Inport  Port=2
  Add : Sum
  Compare To Constant : simulink/Logic and Bit Operations/Compare To Constant  relop=>  const=8  OutDataTypeStr=boolean
  Constant : Constant  Value=2  OutDataTypeStr=single
  Constant1 : Constant  Value=128  OutDataTypeStr=uint8
  Constant2 : Constant  Value=0  OutDataTypeStr=uint8
  Data Type Conversion1 : DataTypeConversion  OutDataTypeStr=uint16  SaturateOnIntegerOverflow=off  RndMeth=Floor
  Data Type Conversion2 : DataTypeConversion  OutDataTypeStr=single  SaturateOnIntegerOverflow=off  RndMeth=Floor
  Display2 : Display
      settings: Format=binary (Stored Integer)
  Divide : Product  Inputs=*/
  Pow : Math  Operator=pow  SignedPower=on  RndMeth=Zero
  Switch : Switch  Threshold=1  SaturateOnIntegerOverflow=off  InputSameDT=off
  Out1 : Outport
  wires:
  Pow/1 -> Data Type Conversion1/1
  Constant/1 -> Pow/1
  In2/1 -> Data Type Conversion2/1
  Data Type Conversion1/1 -> Divide/2
  Data Type Conversion2/1 -> Compare To Constant/1, Pow/2
  Add/1 -> Display2/1, Divide/1
  In1/1 -> Add/2
  Constant1/1 -> Add/1
  Compare To Constant/1 -> Switch/2
  Constant2/1 -> Switch/1
  Divide/1 -> Switch/3
  Switch/1 -> Out1/1

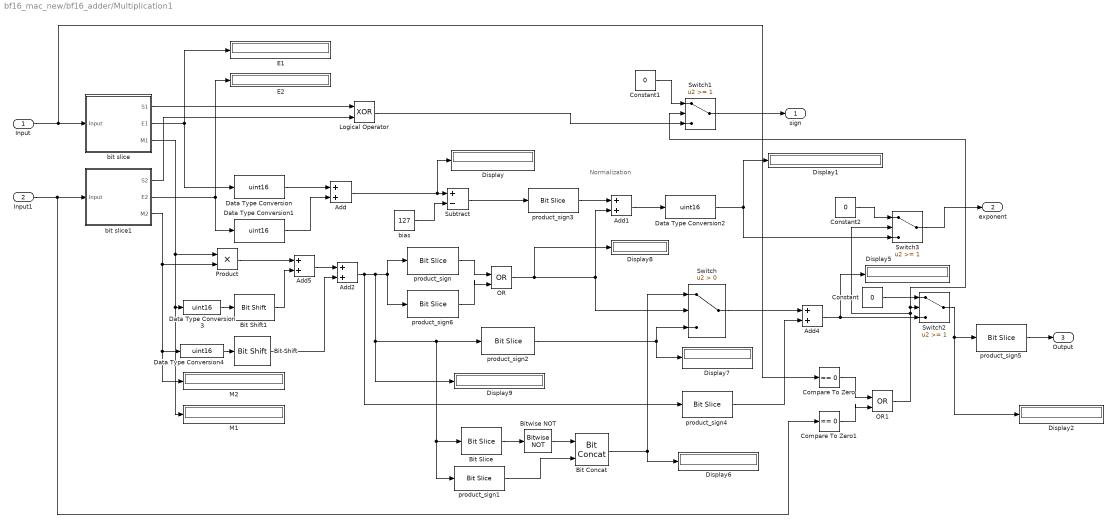
== system bf16_mac_new/bf16_adder/Multiplication1 ==
  note: Normalization
  Input : Inport
  Input1 : Inport  Port=2
  Add{,2,4..5} (4 alike) : Sum  AccumDataTypeStr=uint16
  Add1 : Sum
  Bit Concat : hdlsllib/Logic and Bit Operations/Bit Concat  numInputs=2
  Bit Shift : hdlsllib/Logic and Bit Operations/Bit Shift  mode=Shift Left Logical  N=7
  Bit Shift1 : hdlsllib/Logic and Bit Operations/Bit Shift  mode=Shift Left Logical  N=7
  Bit Slice : hdlsllib/Logic and Bit Operations/Bit Slice  lidx=14  ridx=14
  Bitwise NOT : simulink/Logic and Bit Operations/Bitwise Operator  logicop=NOT  UseBitMask=off  BitMask=bin2dec('11011001')  BitMaskRealWorld=Stored Integer
      settings: LibrarySourceBlock=|
      | simulink/Quick Insert/Logic and Bit
      | Operations/Bitwise NOT
  Compare To Zero : simulink/Logic and Bit Operations/Compare To Zero  relop===  OutDataTypeStr=boolean
  Compare To Zero1 : simulink/Logic and Bit Operations/Compare To Zero  relop===  OutDataTypeStr=boolean
  Constant : Constant  Value=0  OutDataTypeStr=uint8
  Constant1 : Constant  Value=0  OutDataTypeStr=boolean
  Constant2 : Constant  Value=0  OutDataTypeStr=uint16
  Data Type Conversion{,1..4} (5 alike) : DataTypeConversion  OutDataTypeStr=uint16  SaturateOnIntegerOverflow=off  RndMeth=Floor
  Display{,1..2,5..9} (8 alike) : Display
      settings: Format=binary (Stored Integer)
  E1 : Display
      settings: Format=binary (Stored Integer)
  E2 : Display
      settings: Format=binary (Stored Integer)
  Logical Operator : Logic  Operator=XOR  AllPortsSameDT=off  OutDataTypeStr=boolean
  M1 : Display
      settings: Format=binary (Stored Integer)
  M2 : Display
      settings: Format=binary (Stored Integer)
  OR : Logic  Operator=OR  IconShape=distinctive  AllPortsSameDT=off  OutDataTypeStr=boolean
  OR1 : Logic  Operator=OR  IconShape=distinctive  AllPortsSameDT=off  OutDataTypeStr=boolean
  Product : Product  OutDataTypeStr=uint16
  Subtract : Sum  Inputs=+-
  Switch : Switch  Criteria=u2 > Threshold  SaturateOnIntegerOverflow=off  InputSameDT=off
  Switch1 : Switch  Threshold=1  SaturateOnIntegerOverflow=off  InputSameDT=off
  Switch2 : Switch  Threshold=1  SaturateOnIntegerOverflow=off  InputSameDT=off
  Switch3 : Switch  Threshold=1  SaturateOnIntegerOverflow=off  InputSameDT=off
  bias : Constant  Value=127  OutDataTypeStr=uint16
  bit slice : Subsystem
  bit slice1 : Subsystem
  product_sign : hdlsllib/Logic and Bit Operations/Bit Slice  lidx=15  ridx=15
  product_sign1 : hdlsllib/Logic and Bit Operations/Bit Slice  lidx=13  ridx=7
  product_sign2 : hdlsllib/Logic and Bit Operations/Bit Slice  lidx=13  ridx=6
  product_sign3 : hdlsllib/Logic and Bit Operations/Bit Slice  lidx=7  ridx=0
  product_sign4 : hdlsllib/Logic and Bit Operations/Bit Slice  lidx=0  ridx=0
  product_sign5 : hdlsllib/Logic and Bit Operations/Bit Slice  lidx=7  ridx=1
  product_sign6 : hdlsllib/Logic and Bit Operations/Bit Slice  lidx=14  ridx=14
  sign : Outport
  exponent : Outport  Port=2
  Output : Outport  Port=3
  wires:
  Input/1 -> Compare To Zero/1, bit slice/1(Input)
  Input1/1 -> Compare To Zero1/1, bit slice1/1(Input)
  bit slice/1(S1) -> Logical Operator/1
  bit slice1/1(S2) -> Logical Operator/2
  bit slice/2(E1) -> Data Type Conversion/1, E1/1
  bit slice1/2(E2) -> Data Type Conversion1/1, E2/1
  Add/1 -> Display/1, Subtract/1
  Subtract/1 -> product_sign3/1
  bit slice/3(M1) -> Data Type Conversion3/1, M1/1, Product/1
  bit slice1/3(M2) -> Data Type Conversion4/1, M2/1, Product/2
  product_sign2/1 -> Switch/3, Display7/1
  Add1/1 -> Data Type Conversion2/1
  product_sign3/1 -> Add1/1
  Add2/1 -> product_sign4/1, product_sign1/1, Bit Slice/1, product_sign2/1, Display9/1, product_sign6/1, product_sign/1
  Data Type Conversion2/1 -> Display1/1, Switch3/3
  Data Type Conversion/1 -> Add/1
  Data Type Conversion1/1 -> Add/2
  bias/1 -> Subtract/2
  Add4/1 -> Display5/1, Switch2/3
  product_sign4/1 -> Add4/2
  Switch/1 -> Add4/1
  Product/1 -> Add5/1
  Add5/1 -> Add2/1
  product_sign5/1 -> Output/1
  Data Type Conversion4/1 -> Bit Shift/1
  Bit Shift/1 -> Add2/2
  Data Type Conversion3/1 -> Bit Shift1/1
  Bit Shift1/1 -> Add5/2
  product_sign/1 -> OR/1
  OR/1 -> Add1/2, Switch/2, Display8/1
  Bit Slice/1 -> Bitwise NOT/1
  Bitwise NOT/1 -> Bit Concat/1
  product_sign1/1 -> Bit Concat/2
  Bit Concat/1 -> Switch/1, Display6/1
  product_sign6/1 -> OR/2
  Switch2/1 -> product_sign5/1, Display2/1
  Compare To Zero/1 -> OR1/1
  Compare To Zero1/1 -> OR1/2
  OR1/1 -> Switch1/2, Switch2/2, Switch3/2
  Constant/1 -> Switch2/1
  Switch1/1 -> sign/1
  Constant1/1 -> Switch1/1
  Logical Operator/1 -> Switch1/3
  Switch3/1 -> exponent/1
  Constant2/1 -> Switch3/1

== system bf16_mac_new/bf16_adder/Subsystem ==
  u : Inport
  u1 : Inport  Port=2
  u3 : Inport  Port=3
  Bit Concat1 : hdlsllib/Logic and Bit Operations/Bit Concat  numInputs=3
  Extract Sign6 : hdlsllib/Logic and Bit Operations/Bit Slice  lidx=7  ridx=0
  Extract Sign7 : hdlsllib/Logic and Bit Operations/Bit Slice  lidx=0  ridx=0
  y : Outport
  wires:
  u/1 -> Extract Sign7/1
  u3/1 -> Bit Concat1/3
  Extract Sign7/1 -> Bit Concat1/1  "sign"
  Extract Sign6/1 -> Bit Concat1/2  "sign"
  u1/1 -> Extract Sign6/1
  Bit Concat1/1 -> y/1

== system bf16_mac_new/bf16_adder/Subsystem1 ==
  u : Inport
  u1 : Inport  Port=2
  u3 : Inport  Port=3
  Bit Concat1 : hdlsllib/Logic and Bit Operations/Bit Concat  numInputs=3
  Extract Sign6 : hdlsllib/Logic and Bit Operations/Bit Slice  lidx=7  ridx=0
  Extract Sign7 : hdlsllib/Logic and Bit Operations/Bit Slice  lidx=0  ridx=0
  y : Outport
  wires:
  u/1 -> Extract Sign7/1
  u3/1 -> Bit Concat1/3
  Extract Sign7/1 -> Bit Concat1/1  "sign"
  Extract Sign6/1 -> Bit Concat1/2  "sign"
  u1/1 -> Extract Sign6/1
  Bit Concat1/1 -> y/1

== system bf16_mac_new/bf16_adder/Subsystem2 ==
  u : Inport
  u1 : Inport  Port=2
  u3 : Inport  Port=3
  Bit Concat1 : hdlsllib/Logic and Bit Operations/Bit Concat  numInputs=3
  Extract Sign6 : hdlsllib/Logic and Bit Operations/Bit Slice  lidx=7  ridx=0
  Extract Sign7 : hdlsllib/Logic and Bit Operations/Bit Slice  lidx=0  ridx=0
  y : Outport
  wires:
  u/1 -> Extract Sign7/1
  u3/1 -> Bit Concat1/3
  Extract Sign7/1 -> Bit Concat1/1  "sign"
  Extract Sign6/1 -> Bit Concat1/2  "sign"
  u1/1 -> Extract Sign6/1
  Bit Concat1/1 -> y/1

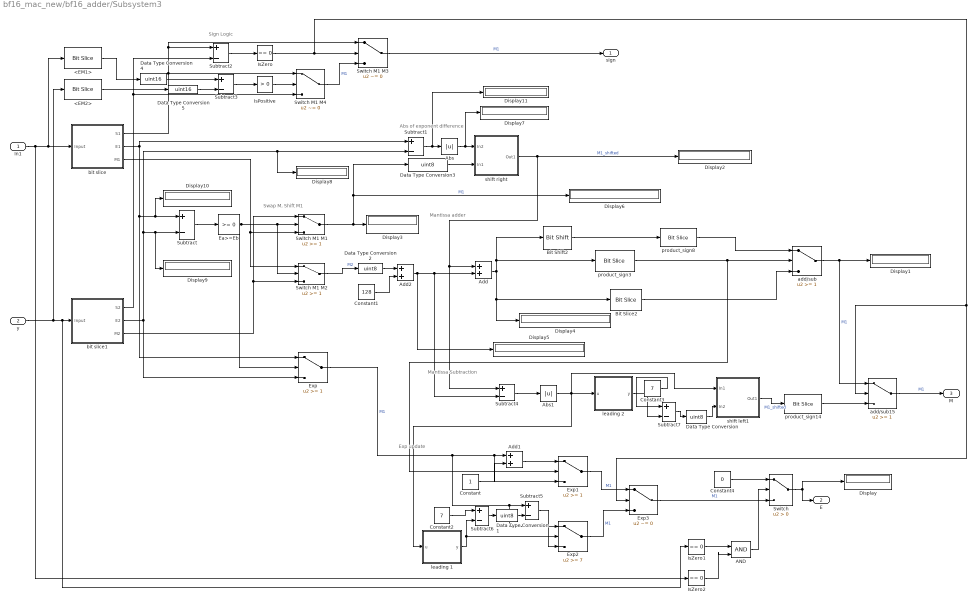
== system bf16_mac_new/bf16_adder/Subsystem3 ==
  note: Mantissa Subtraction
  note: Exp update
  note: Mantissa adder
  note: Sign Logic
  note: Abs of exponent difference
  note: Swap M, Shift M1
  In1 : Inport
  y : Inport  Port=2
  <EM1> : hdlsllib/Logic and Bit Operations/Bit Slice  lidx=14  ridx=0
  <EM2> : hdlsllib/Logic and Bit Operations/Bit Slice  lidx=14  ridx=0
  AND : Logic  IconShape=distinctive  AllPortsSameDT=off  OutDataTypeStr=boolean
  Abs : Abs  SaturateOnIntegerOverflow=off
  Abs1 : Abs  SaturateOnIntegerOverflow=off
  Add : Sum  OutDataTypeStr=uint16
  Add1 : Sum
  Add2 : Sum
  Bit Shift2 : hdlsllib/Logic and Bit Operations/Bit Shift  mode=Shift Right Logical  N=1
  Bit Slice2 : hdlsllib/Logic and Bit Operations/Bit Slice  lidx=6  ridx=0
  Constant : Constant  OutDataTypeStr=uint8  SampleTime=-1
  Constant1 : Constant  Value=128  OutDataTypeStr=uint8  SampleTime=-1
  Constant2 : Constant  Value=7  SampleTime=-1
  Constant3 : Constant  Value=7  SampleTime=-1
  Constant4 : Constant  Value=0  OutDataTypeStr=uint8  SampleTime=-1
  Data Type Conversion{,1..3} (4 alike) : DataTypeConversion  OutDataTypeStr=uint8  SaturateOnIntegerOverflow=off  RndMeth=Floor
  Data Type Conversion4 : DataTypeConversion  OutDataTypeStr=uint16  SaturateOnIntegerOverflow=off  RndMeth=Floor
  Data Type Conversion5 : DataTypeConversion  OutDataTypeStr=uint16  SaturateOnIntegerOverflow=off  RndMeth=Floor
  Display{,1..11} (12 alike) : Display
      Display settings: Format=binary (Stored Integer)
      Display1 settings: Format=binary (Stored Integer)
      Display10 settings: Format=binary (Stored Integer)
      Display11 settings: Format=decimal (Stored Integer)
      Display2 settings: Format=binary (Stored Integer)
      Display3 settings: Format=binary (Stored Integer)
      Display4 settings: Format=binary (Stored Integer)
      Display5 settings: Format=binary (Stored Integer)
      Display6 settings: Format=binary (Stored Integer)
      Display7 settings: Format=decimal (Stored Integer)
      Display8 settings: Format=binary (Stored Integer)
      Display9 settings: Format=binary (Stored Integer)
  Ea>=Eb : hdlsllib/Logic and Bit Operations/Compare To Zero  relop=>=  OutDataTypeStr=boolean
  Exp : Switch  Threshold=1  SaturateOnIntegerOverflow=off  InputSameDT=off
  Exp1 : Switch  Threshold=1  SaturateOnIntegerOverflow=off  InputSameDT=off
  Exp2 : Switch  Threshold=7  SaturateOnIntegerOverflow=off  InputSameDT=off
  Exp3 : Switch  Criteria=u2 ~= 0  Threshold=1  SaturateOnIntegerOverflow=off  InputSameDT=off
  IsPositive : simulink/Logic and Bit Operations/Compare To Zero  relop=>  OutDataTypeStr=boolean
      settings: LibrarySourceBlock=|
      | simulink/Quick Insert/Logic and Bit
      | Operations/IsPositive
  IsZero : simulink/Logic and Bit Operations/Compare To Zero  relop===  OutDataTypeStr=boolean
      settings: LibrarySourceBlock=|
      | simulink/Quick Insert/Logic and Bit
      | Operations/IsZero
  IsZero1 : simulink/Logic and Bit Operations/Compare To Zero  relop===  OutDataTypeStr=boolean
      settings: LibrarySourceBlock=|
      | simulink/Quick Insert/Logic and Bit
      | Operations/IsZero
  IsZero2 : simulink/Logic and Bit Operations/Compare To Zero  relop===  OutDataTypeStr=boolean
      settings: LibrarySourceBlock=|
      | simulink/Quick Insert/Logic and Bit
      | Operations/IsZero
  Subtract{,1,3..4} (4 alike) : Sum  Inputs=+-  OutDataTypeStr=int16
  Subtract2 : Sum  Inputs=+-  OutDataTypeStr=int8
  Subtract5 : Sum  Inputs=+-  OutDataTypeStr=uint8
  Subtract6 : Sum  Inputs=+-
  Subtract7 : Sum  Inputs=+-
  Switch : Switch  Criteria=u2 > Threshold  SaturateOnIntegerOverflow=off  InputSameDT=off
  Switch M1 M1 : Switch  Threshold=1  SaturateOnIntegerOverflow=off  InputSameDT=off
  Switch M1 M2 : Switch  Threshold=1  SaturateOnIntegerOverflow=off  InputSameDT=off
  Switch M1 M3 : Switch  Criteria=u2 ~= 0  Threshold=1  SaturateOnIntegerOverflow=off  InputSameDT=off
  Switch M1 M4 : Switch  Criteria=u2 ~= 0  Threshold=1  SaturateOnIntegerOverflow=off  InputSameDT=off
  add/sub : Switch  Threshold=1  SaturateOnIntegerOverflow=off  InputSameDT=off
  add/sub15 : Switch  Threshold=1  SaturateOnIntegerOverflow=off  InputSameDT=off
  bit slice : Subsystem
  bit slice1 : Subsystem
  leading 1 : Subsystem
  leading 2 : Subsystem
  product_sign14 : hdlsllib/Logic and Bit Operations/Bit Slice  lidx=6  ridx=0
  product_sign3 : hdlsllib/Logic and Bit Operations/Bit Slice  lidx=8  ridx=8
  product_sign8 : hdlsllib/Logic and Bit Operations/Bit Slice  lidx=6  ridx=0
  shift left1 : Subsystem
  shift right : Subsystem
  sign : Outport
  E : Outport  Port=2
  M : Outport  Port=3
  wires:
  In1/1 -> bit slice/1(Input), <EM1>/1, IsZero2/1
  Subtract/1 -> Ea>=Eb/1
  Ea>=Eb/1 -> Exp/2, Switch M1 M2/2, Switch M1 M1/2
  bit slice/3(M1) -> Switch M1 M1/3, Switch M1 M2/1
  bit slice1/3(M2) -> Switch M1 M2/3, Switch M1 M1/1
  Switch M1 M1/1 -> Display6/1, Data Type Conversion3/1, Display3/1  "M1"
  Subtract1/1 -> Display11/1, Abs/1
  bit slice1/1(S2) -> Switch M1 M4/3, Subtract2/2
  bit slice/1(S1) -> Switch M1 M4/1, Subtract2/1, Switch M1 M3/1
  Subtract2/1 -> IsZero/1
  IsZero/1 -> add/sub15/2, Exp3/2, Switch M1 M3/2
  Abs/1 -> Display7/1, shift right/1(In2)
  shift right/1(Out1) -> Subtract4/1, Add/1, Display2/1  "M1_shifted"
  IsPositive/1 -> Switch M1 M4/2
  Switch M1 M4/1 -> Switch M1 M3/3  "M1"
  Switch M1 M3/1 -> sign/1  "M1"
  Switch M1 M2/1 -> Data Type Conversion2/1  "M2"
  Subtract3/1 -> IsPositive/1
  <EM1>/1 -> Data Type Conversion4/1
  <EM2>/1 -> Data Type Conversion5/1
  Subtract4/1 -> Abs1/1
  Data Type Conversion3/1 -> shift right/2(In1)
  Data Type Conversion2/1 -> Add2/1
  add/sub/1 -> add/sub15/1, Display1/1  "M1"
  Exp/1 -> Exp2/1, Subtract5/1, Add1/1, Exp1/3  "M1"
  product_sign3/1 -> add/sub/2, Exp1/2
  Constant/1 -> Add1/2
  Add1/1 -> Exp1/1
  Subtract5/1 -> Exp2/3
  Add/1 -> Bit Slice2/1, Display4/1, product_sign3/1, Bit Shift2/1
  Bit Shift2/1 -> product_sign8/1
  Bit Slice2/1 -> add/sub/3
  Add2/1 -> Subtract4/2, Add/2, Display5/1
  Constant1/1 -> Add2/2
  product_sign8/1 -> add/sub/1
  product_sign14/1 -> add/sub15/3
  Exp1/1 -> Exp3/1  "M1"
  Exp2/1 -> Exp3/3  "M1"
  Data Type Conversion4/1 -> Subtract3/1
  Data Type Conversion5/1 -> Subtract3/2
  add/sub15/1 -> M/1  "M1"
  leading 1/1(y) -> Exp2/2, Subtract6/2
  Constant2/1 -> Subtract6/1
  leading 2/1(y) -> Subtract7/2
  Constant3/1 -> Subtract7/1
  Abs1/1 -> leading 1/1(u), shift left1/1(In1), leading 2/1(u)
  shift left1/1(Out1) -> product_sign14/1  "M1_shifted"
  bit slice/2(E1) -> Subtract1/1, Display10/1, Subtract/1, Exp/1
  bit slice1/2(E2) -> Exp/3, Display9/1, Subtract/2, Display8/1, Subtract1/2
  Switch/1 -> E/1, Display/1
  IsZero1/1 -> AND/1
  IsZero2/1 -> AND/2
  AND/1 -> Switch/2
  y/1 -> bit slice1/1(Input), IsZero1/1, <EM2>/1
  Exp3/1 -> Switch/3  "M1"
  Constant4/1 -> Switch/1
  Subtract7/1 -> Data Type Conversion/1
  Data Type Conversion/1 -> shift left1/2(In2)
  Subtract6/1 -> Data Type Conversion1/1
  Data Type Conversion1/1 -> Subtract5/2

== system bf16_mac_new/bf16_adder/Subsystem4 ==
  u : Inport
  u1 : Inport  Port=2
  u3 : Inport  Port=3
  Bit Concat1 : hdlsllib/Logic and Bit Operations/Bit Concat  numInputs=3
  Extract Sign6 : hdlsllib/Logic and Bit Operations/Bit Slice  lidx=7  ridx=0
  Extract Sign7 : hdlsllib/Logic and Bit Operations/Bit Slice  lidx=0  ridx=0
  y : Outport
  wires:
  u/1 -> Extract Sign7/1
  u3/1 -> Bit Concat1/3
  Extract Sign7/1 -> Bit Concat1/1  "sign"
  Extract Sign6/1 -> Bit Concat1/2  "sign"
  u1/1 -> Extract Sign6/1
  Bit Concat1/1 -> y/1

== system bf16_mac_new/bf16_adder/bit slice ==
  Input : Inport
  Display : Display
      settings: Format=binary (Stored Integer)
  Extract Exponent : hdlsllib/Logic and Bit Operations/Bit Slice  lidx=14  ridx=7
  Extract Mantissa : hdlsllib/Logic and Bit Operations/Bit Slice  lidx=6  ridx=0
  Extract Sign : hdlsllib/Logic and Bit Operations/Bit Slice  lidx=15  ridx=15
  S1 : Outport
  E1 : Outport  Port=2
  M1 : Outport  Port=3
  wires:
  Input/1 -> Extract Mantissa/1, Extract Exponent/1, Extract Sign/1, Display/1
  Extract Mantissa/1 -> M1/1  "mantissa"
  Extract Sign/1 -> S1/1  "sign"
  Extract Exponent/1 -> E1/1

== system bf16_mac_new/bf16_adder/bit slice1 ==
  Input : Inport
  Display : Display
      settings: Format=binary (Stored Integer)
  Extract Exponent : hdlsllib/Logic and Bit Operations/Bit Slice  lidx=14  ridx=7
  Extract Mantissa : hdlsllib/Logic and Bit Operations/Bit Slice  lidx=6  ridx=0
  Extract Sign : hdlsllib/Logic and Bit Operations/Bit Slice  lidx=15  ridx=15
  S2 : Outport
  E2 : Outport  Port=2
  M2 : Outport  Port=3
  wires:
  Input/1 -> Extract Mantissa/1, Extract Exponent/1, Extract Sign/1, Display/1
  Extract Mantissa/1 -> M2/1  "mantissa"
  Extract Sign/1 -> S2/1  "sign"
  Extract Exponent/1 -> E2/1

== system bf16_mac_new/bf16_adder/bit slice2 ==
  Input : Inport
  Display : Display
      settings: Format=binary (Stored Integer)
  Extract Exponent : hdlsllib/Logic and Bit Operations/Bit Slice  lidx=14  ridx=7
  Extract Mantissa : hdlsllib/Logic and Bit Operations/Bit Slice  lidx=6  ridx=0
  Extract Sign : hdlsllib/Logic and Bit Operations/Bit Slice  lidx=15  ridx=15
  S1 : Outport
  E1 : Outport  Port=2
  M1 : Outport  Port=3
  wires:
  Input/1 -> Extract Mantissa/1, Extract Exponent/1, Extract Sign/1, Display/1
  Extract Mantissa/1 -> M1/1  "mantissa"
  Extract Sign/1 -> S1/1  "sign"
  Extract Exponent/1 -> E1/1

== system bf16_mac_new/bf16_adder/bit slice3 ==
  Input : Inport
  Display : Display
      settings: Format=binary (Stored Integer)
  Extract Exponent : hdlsllib/Logic and Bit Operations/Bit Slice  lidx=14  ridx=7
  Extract Mantissa : hdlsllib/Logic and Bit Operations/Bit Slice  lidx=6  ridx=0
  Extract Sign : hdlsllib/Logic and Bit Operations/Bit Slice  lidx=15  ridx=15
  S2 : Outport
  E2 : Outport  Port=2
  M2 : Outport  Port=3
  wires:
  Input/1 -> Extract Mantissa/1, Extract Exponent/1, Extract Sign/1, Display/1
  Extract Mantissa/1 -> M2/1  "mantissa"
  Extract Sign/1 -> S2/1  "sign"
  Extract Exponent/1 -> E2/1

== system bf16_mac_new/bf16_adder/leading 1 ==
  u : Inport
  MATLAB Function : MATLAB Function  TreatAsAtomicUnit=on
  y : Outport
  wires:
  u/1 -> MATLAB Function/1(u)
  MATLAB Function/1(y) -> y/1
